simulink model "Thirtybussys"  (R2023b)
settings: Solver=VariableStepAuto  StartTime=0.0  StopTime=1  RelTol=1e-3
libraries: spsFourierLib x60, spsThreePhaseSeriesRLCBranchLib x41, spsThreePhaseVIMeasurementLib x30, spsPower3phInstantaneousLib x30, spsThreePhaseSeriesRLCLoadLib x21, spsThreePhaseSourceLib x6, spsThreePhaseTransformerTwoWindingsLib x6, spsThreePhaseFaultLib x1, sps_lib x1
(part 1 of 2)
settings Model: Creator=sariy sh  LastModifiedBy=HP
settings SolverCC: AlgebraicLoopSolver=TrustRegion
settings DataIOCC: ReturnWorkspaceOutputs=off
settings DebuggingCC: UnconnectedInputMsg=warning  UnconnectedOutputMsg=warning  UnconnectedLineMsg=warning  ArithmeticOperatorsInVariantConditions=warning
settings ModelReferenceCC: EnableRefExpFcnMdlSchedulingChecks=on
settings SFSimCC: SimUseLocalCustomCode=off  CustomCodeUndefinedFunction=UseInterfaceOnly
settings RTWCC: RTWUseLocalCustomCode=off
settings CodeAppCC: StateflowObjectComments=on
settings SimscapeCC: SimscapeNormalizeSystem=off

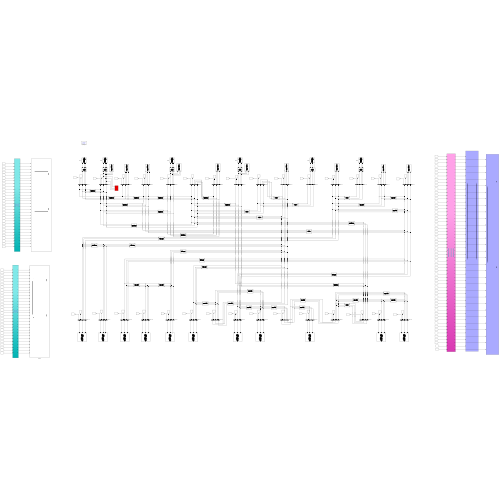
[thumbnail: Simulink's stored preview of the top-level diagram]
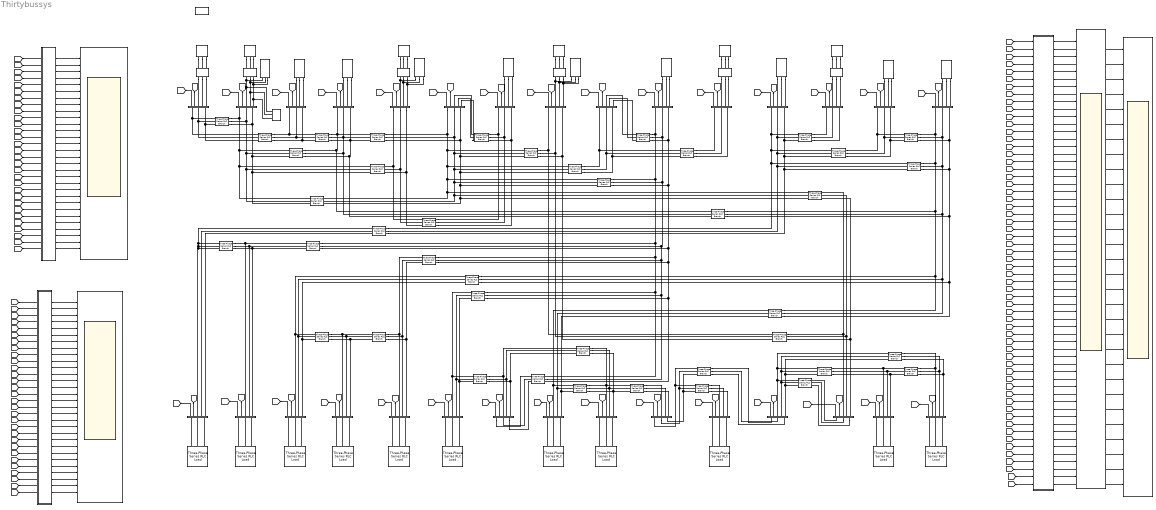
== system Thirtybussys ==
  Bus {1..30} (30 alike) : spsThreePhaseVIMeasurementLib/Three-Phase V-I Measurement  VoltageMeasurement=phase-to-ground  SetLabelV=off  LabelV=Vabc  Vpu=off  VpuLL=off  CurrentMeasurement=yes  SetLabelI=off  LabelI=Iabc  Ipu=off  Pbase=100e6  Vbase=500e3  OutputType=Complex  PhasorSimulation=off  PSBequivalent=0
  Gen1 : spsThreePhaseSourceLib/Three-Phase Source  InternalConnection=Yg  VoltagePhases=off  Voltage=1.06  PhaseAngle=0  Voltage_phases=[25e3 25e3 25e3]/sqrt(3)  PhaseAngles_phases=[0 -120 +120]  Frequency=50  NonIdealSource=on  SpecifyImpedance=on  Resistance=0.8929  Inductance=16.58e-3  ShortCircuitLevel=100e6  BaseVoltage=1  XRratio=1  BusType=swing  Pref=10e3  Qref=0  Prefabc=[10e3, 10e3, 10e3]  Qrefabc=[0, 0, 0]  Qmin=-inf  Qmax=inf
  Gen2 : spsThreePhaseSourceLib/Three-Phase Source  InternalConnection=Yg  VoltagePhases=off  Voltage=1.045  PhaseAngle=0  Voltage_phases=[25e3 25e3 25e3]/sqrt(3)  PhaseAngles_phases=[0 -120 +120]  Frequency=50  NonIdealSource=on  SpecifyImpedance=on  Resistance=0.8929  Inductance=16.58e-3  ShortCircuitLevel=100e6  BaseVoltage=1  XRratio=1  BusType=PQ  Pref=0.4  Qref=0.5  Prefabc=[10e3, 10e3, 10e3]  Qrefabc=[0, 0, 0]  Qmin=-inf  Qmax=inf
  Gen3 : spsThreePhaseSourceLib/Three-Phase Source  InternalConnection=Yg  VoltagePhases=off  Voltage=1.010  PhaseAngle=0  Voltage_phases=[25e3 25e3 25e3]/sqrt(3)  PhaseAngles_phases=[0 -120 +120]  Frequency=50  NonIdealSource=on  SpecifyImpedance=on  Resistance=0.8929  Inductance=16.58e-3  ShortCircuitLevel=100e6  BaseVoltage=1  XRratio=1  BusType=PV  Pref=0.37  Qref=0  Prefabc=[10e3, 10e3, 10e3]  Qrefabc=[0, 0, 0]  Qmin=-0.15  Qmax=0.625
  Gen4 : spsThreePhaseSourceLib/Three-Phase Source  InternalConnection=Yg  VoltagePhases=off  Voltage=1.010  PhaseAngle=0  Voltage_phases=[25e3 25e3 25e3]/sqrt(3)  PhaseAngles_phases=[0 -120 +120]  Frequency=50  NonIdealSource=on  SpecifyImpedance=on  Resistance=0.8929  Inductance=16.58e-3  ShortCircuitLevel=100e6  BaseVoltage=1  XRratio=1  BusType=PV  Pref=0.373  Qref=0  Prefabc=[10e3, 10e3, 10e3]  Qrefabc=[0, 0, 0]  Qmin=-0.15  Qmax=0.50
  Gen5 : spsThreePhaseSourceLib/Three-Phase Source  InternalConnection=Yg  VoltagePhases=off  Voltage=1.082  PhaseAngle=0  Voltage_phases=[25e3 25e3 25e3]/sqrt(3)  PhaseAngles_phases=[0 -120 +120]  Frequency=50  NonIdealSource=on  SpecifyImpedance=on  Resistance=0.8929  Inductance=16.58e-3  ShortCircuitLevel=100e6  BaseVoltage=1  XRratio=1  BusType=PV  Pref=0.162  Qref=0  Prefabc=[10e3, 10e3, 10e3]  Qrefabc=[0, 0, 0]  Qmin=-0.10  Qmax=0.40
  Gen6 : spsThreePhaseSourceLib/Three-Phase Source  InternalConnection=Yg  VoltagePhases=off  Voltage=1.071  PhaseAngle=0  Voltage_phases=[25e3 25e3 25e3]/sqrt(3)  PhaseAngles_phases=[0 -120 +120]  Frequency=50  NonIdealSource=on  SpecifyImpedance=on  Resistance=0.8929  Inductance=16.58e-3  ShortCircuitLevel=100e6  BaseVoltage=1  XRratio=1  BusType=PV  Pref=0.106  Qref=0  Prefabc=[10e3, 10e3, 10e3]  Qrefabc=[0, 0, 0]  Qmin=-0.15  Qmax=0.45
  Scope{,1..3} (4 alike) : Scope  NumInputPorts=30
  Subsystem : Subsystem
  Subsystem1 : Subsystem
  Subsystem30 : Subsystem
  Three-Phase Series RLC Branch : spsThreePhaseSeriesRLCBranchLib/Three-Phase Series RLC Branch  LConnTagsString=A|B|C  RConnTagsString=A|B|C  BranchType=RLC  Resistance=0.0192  Inductance=0.0575/(2*pi*50)  Capacitance=1/0.0264/(2*pi*50)  Measurements=None
  Three-Phase Series RLC Branch1 : spsThreePhaseSeriesRLCBranchLib/Three-Phase Series RLC Branch  LConnTagsString=A|B|C  RConnTagsString=A|B|C  BranchType=RLC  Resistance=0.0452  Inductance=0.1652/(2*pi*50)  Capacitance=1/0.0204/(2*pi*50)  Measurements=None
  Three-Phase Series RLC Branch10 : spsThreePhaseSeriesRLCBranchLib/Three-Phase Series RLC Branch  LConnTagsString=A|B|C  RConnTagsString=A|B|C  BranchType=L  Resistance=0  Inductance=0.2080/(2*pi*50)  Capacitance=0  Measurements=None
  Three-Phase Series RLC Branch11 : spsThreePhaseSeriesRLCBranchLib/Three-Phase Series RLC Branch  LConnTagsString=A|B|C  RConnTagsString=A|B|C  BranchType=L  Resistance=1  Inductance=0.1100/(2*pi*50)  Capacitance=1e-6  Measurements=None
  Three-Phase Series RLC Branch12 : spsThreePhaseSeriesRLCBranchLib/Three-Phase Series RLC Branch  LConnTagsString=A|B|C  RConnTagsString=A|B|C  BranchType=L  Resistance=1  Inductance=0.5560/(2*pi*50)  Capacitance=1e-6  Measurements=None
  Three-Phase Series RLC Branch13 : spsThreePhaseSeriesRLCBranchLib/Three-Phase Series RLC Branch  LConnTagsString=A|B|C  RConnTagsString=A|B|C  BranchType=L  Resistance=1  Inductance=0.2080/(2*pi*50)  Capacitance=1e-6  Measurements=None
  Three-Phase Series RLC Branch14 : spsThreePhaseSeriesRLCBranchLib/Three-Phase Series RLC Branch  LConnTagsString=A|B|C  RConnTagsString=A|B|C  BranchType=L  Resistance=1  Inductance=0.1400/(2*pi*50)  Capacitance=1e-6  Measurements=None
  Three-Phase Series RLC Branch15 : spsThreePhaseSeriesRLCBranchLib/Three-Phase Series RLC Branch  LConnTagsString=A|B|C  RConnTagsString=A|B|C  BranchType=RL  Resistance=0.1231  Inductance=0.2559/(2*pi*50)  Capacitance=1e-6  Measurements=None
  Three-Phase Series RLC Branch16 : spsThreePhaseSeriesRLCBranchLib/Three-Phase Series RLC Branch  LConnTagsString=A|B|C  RConnTagsString=A|B|C  BranchType=RL  Resistance=0.2210  Inductance=0.1997/(2*pi*50)  Capacitance=1e-6  Measurements=None
  Three-Phase Series RLC Branch17 : spsThreePhaseSeriesRLCBranchLib/Three-Phase Series RLC Branch  LConnTagsString=A|B|C  RConnTagsString=A|B|C  BranchType=L  Resistance=1  Inductance=0.2560/(2*pi*50)  Capacitance=1e-6  Measurements=None
  Three-Phase Series RLC Branch18 : spsThreePhaseSeriesRLCBranchLib/Three-Phase Series RLC Branch  LConnTagsString=A|B|C  RConnTagsString=A|B|C  BranchType=RL  Resistance=0.0945  Inductance=0.1987/(2*pi*50)  Capacitance=1e-6  Measurements=None
  Three-Phase Series RLC Branch19 : spsThreePhaseSeriesRLCBranchLib/Three-Phase Series RLC Branch  LConnTagsString=A|B|C  RConnTagsString=A|B|C  BranchType=RLC  Resistance=0.0524  Inductance=0.1923/(2*pi*50)  Capacitance=1e-6  Measurements=None
  Three-Phase Series RLC Branch2 : spsThreePhaseSeriesRLCBranchLib/Three-Phase Series RLC Branch  LConnTagsString=A|B|C  RConnTagsString=A|B|C  BranchType=RLC  Resistance=0.0132  Inductance=0.0379/(2*pi*50)  Capacitance=1/0.0042/(2*pi*50)  Measurements=None
  Three-Phase Series RLC Branch20 : spsThreePhaseSeriesRLCBranchLib/Three-Phase Series RLC Branch  LConnTagsString=A|B|C  RConnTagsString=A|B|C  BranchType=RL  Resistance=0.0324  Inductance=0.0845/(2*pi*50)  Capacitance=1e-6  Measurements=None
  Three-Phase Series RLC Branch21 : spsThreePhaseSeriesRLCBranchLib/Three-Phase Series RLC Branch  LConnTagsString=A|B|C  RConnTagsString=A|B|C  BranchType=RL  Resistance=0.1063  Inductance=0.2185/(2*pi*50)  Capacitance=1e-6  Measurements=None
  Three-Phase Series RLC Branch22 : spsThreePhaseSeriesRLCBranchLib/Three-Phase Series RLC Branch  LConnTagsString=A|B|C  RConnTagsString=A|B|C  BranchType=RL  Resistance=0.0639  Inductance=0.1292/(2*pi*50)  Capacitance=1e-6  Measurements=None
  Three-Phase Series RLC Branch23 : spsThreePhaseSeriesRLCBranchLib/Three-Phase Series RLC Branch  LConnTagsString=A|B|C  RConnTagsString=A|B|C  BranchType=RL  Resistance=0.0340  Inductance=0.0680/(2*pi*50)  Capacitance=1e-6  Measurements=None
  Three-Phase Series RLC Branch24 : spsThreePhaseSeriesRLCBranchLib/Three-Phase Series RLC Branch  LConnTagsString=A|B|C  RConnTagsString=A|B|C  BranchType=RL  Resistance=0.0936  Inductance=0.2090/(2*pi*50)  Capacitance=1e-6  Measurements=None
  Three-Phase Series RLC Branch25 : spsThreePhaseSeriesRLCBranchLib/Three-Phase Series RLC Branch  LConnTagsString=A|B|C  RConnTagsString=A|B|C  BranchType=RL  Resistance=0.0348  Inductance=0.0749/(2*pi*50)  Capacitance=1e-6  Measurements=None
  Three-Phase Series RLC Branch26 : spsThreePhaseSeriesRLCBranchLib/Three-Phase Series RLC Branch  LConnTagsString=A|B|C  RConnTagsString=A|B|C  BranchType=RL  Resistance=0.0116  Inductance=0.0236/(2*pi*50)  Capacitance=1e-6  Measurements=None
  Three-Phase Series RLC Branch27 : spsThreePhaseSeriesRLCBranchLib/Three-Phase Series RLC Branch  LConnTagsString=A|B|C  RConnTagsString=A|B|C  BranchType=RL  Resistance=0.0727  Inductance=0.1499/(2*pi*50)  Capacitance=1e-6  Measurements=None
  Three-Phase Series RLC Branch28 : spsThreePhaseSeriesRLCBranchLib/Three-Phase Series RLC Branch  LConnTagsString=A|B|C  RConnTagsString=A|B|C  BranchType=RL  Resistance=0.1000  Inductance=0.2020/(2*pi*50)  Capacitance=1e-6  Measurements=None
  Three-Phase Series RLC Branch29 : spsThreePhaseSeriesRLCBranchLib/Three-Phase Series RLC Branch  LConnTagsString=A|B|C  RConnTagsString=A|B|C  BranchType=RL  Resistance=0.1150  Inductance=0.1790/(2*pi*50)  Capacitance=1e-6  Measurements=None
  Three-Phase Series RLC Branch3 : spsThreePhaseSeriesRLCBranchLib/Three-Phase Series RLC Branch  LConnTagsString=A|B|C  RConnTagsString=A|B|C  BranchType=RLC  Resistance=0.0570  Inductance=0.1737/(2*pi*50)  Capacitance=1/0.0184/(2*pi*50)  Measurements=None
  Three-Phase Series RLC Branch30 : spsThreePhaseSeriesRLCBranchLib/Three-Phase Series RLC Branch  LConnTagsString=A|B|C  RConnTagsString=A|B|C  BranchType=RL  Resistance=0.1320  Inductance=0.2700/(2*pi*50)  Capacitance=1e-6  Measurements=None
  Three-Phase Series RLC Branch31 : spsThreePhaseSeriesRLCBranchLib/Three-Phase Series RLC Branch  LConnTagsString=A|B|C  RConnTagsString=A|B|C  BranchType=RL  Resistance=0.1885  Inductance=0.3292/(2*pi*50)  Capacitance=1e-6  Measurements=None
  Three-Phase Series RLC Branch32 : spsThreePhaseSeriesRLCBranchLib/Three-Phase Series RLC Branch  LConnTagsString=A|B|C  RConnTagsString=A|B|C  BranchType=RL  Resistance=0.2544  Inductance=0.3800/(2*pi*50)  Capacitance=1e-6  Measurements=None
  Three-Phase Series RLC Branch33 : spsThreePhaseSeriesRLCBranchLib/Three-Phase Series RLC Branch  LConnTagsString=A|B|C  RConnTagsString=A|B|C  BranchType=RL  Resistance=0.1093  Inductance=0.2087/(2*pi*50)  Capacitance=1e-6  Measurements=None
  Three-Phase Series RLC Branch34 : spsThreePhaseSeriesRLCBranchLib/Three-Phase Series RLC Branch  LConnTagsString=A|B|C  RConnTagsString=A|B|C  BranchType=RL  Resistance=0.2198  Inductance=0.4153/(2*pi*50)  Capacitance=1e-6  Measurements=None
  Three-Phase Series RLC Branch35 : spsThreePhaseSeriesRLCBranchLib/Three-Phase Series RLC Branch  LConnTagsString=A|B|C  RConnTagsString=A|B|C  BranchType=RL  Resistance=0.3202  Inductance=0.6027/(2*pi*50)  Capacitance=1e-6  Measurements=None
  Three-Phase Series RLC Branch36 : spsThreePhaseSeriesRLCBranchLib/Three-Phase Series RLC Branch  LConnTagsString=A|B|C  RConnTagsString=A|B|C  BranchType=L  Resistance=1  Inductance=0.3960/(2*pi*50)  Capacitance=1e-6  Measurements=None
  Three-Phase Series RLC Branch37 : spsThreePhaseSeriesRLCBranchLib/Three-Phase Series RLC Branch  LConnTagsString=A|B|C  RConnTagsString=A|B|C  BranchType=RLC  Resistance=0.0169  Inductance=0.0599/(2*pi*50)  Capacitance=1/0.0065/(2*pi*50)  Measurements=None
  Three-Phase Series RLC Branch38 : spsThreePhaseSeriesRLCBranchLib/Three-Phase Series RLC Branch  LConnTagsString=A|B|C  RConnTagsString=A|B|C  BranchType=RLC  Resistance=0.0636  Inductance=0.2000/(2*pi*50)  Capacitance=1/0.0214/(2*pi*50)  Measurements=None
  Three-Phase Series RLC Branch39 : spsThreePhaseSeriesRLCBranchLib/Three-Phase Series RLC Branch  LConnTagsString=A|B|C  RConnTagsString=A|B|C  BranchType=RL  Resistance=0.0662  Inductance=0.1304/(2*pi*50)  Capacitance=1e-6  Measurements=None
  Three-Phase Series RLC Branch4 : spsThreePhaseSeriesRLCBranchLib/Three-Phase Series RLC Branch  LConnTagsString=A|B|C  RConnTagsString=A|B|C  BranchType=RLC  Resistance=0.0472  Inductance=0.1983/(2*pi*50)  Capacitance=1/0.0209/(2*pi*50)  Measurements=None
  Three-Phase Series RLC Branch40 : spsThreePhaseSeriesRLCBranchLib/Three-Phase Series RLC Branch  LConnTagsString=A|B|C  RConnTagsString=A|B|C  BranchType=RL  Resistance=0.2399  Inductance=0.4533/(2*pi*50)  Capacitance=1e-6  Measurements=None
  Three-Phase Series RLC Branch5 : spsThreePhaseSeriesRLCBranchLib/Three-Phase Series RLC Branch  LConnTagsString=A|B|C  RConnTagsString=A|B|C  BranchType=RLC  Resistance=0.0581  Inductance=0.1763/(2*pi*50)  Capacitance=1/0.0187/(2*pi*50)  Measurements=None
  Three-Phase Series RLC Branch6 : spsThreePhaseSeriesRLCBranchLib/Three-Phase Series RLC Branch  LConnTagsString=A|B|C  RConnTagsString=A|B|C  BranchType=RLC  Resistance=0.0119  Inductance=0.0414/(2*pi*50)  Capacitance=1/0.0045/(2*pi*50)  Measurements=None
  Three-Phase Series RLC Branch7 : spsThreePhaseSeriesRLCBranchLib/Three-Phase Series RLC Branch  LConnTagsString=A|B|C  RConnTagsString=A|B|C  BranchType=RLC  Resistance=0.0267  Inductance=0.0820/(2*pi*50)  Capacitance=1/0.0085/(2*pi*50)  Measurements=None
  Three-Phase Series RLC Branch8 : spsThreePhaseSeriesRLCBranchLib/Three-Phase Series RLC Branch  LConnTagsString=A|B|C  RConnTagsString=A|B|C  BranchType=RLC  Resistance=0.0460  Inductance=0.1160/(2*pi*50)  Capacitance=1/0.0102/(2*pi*50)  Measurements=None
  Three-Phase Series RLC Branch9 : spsThreePhaseSeriesRLCBranchLib/Three-Phase Series RLC Branch  LConnTagsString=A|B|C  RConnTagsString=A|B|C  BranchType=RLC  Resistance=0.0120  Inductance=0.0420/(2*pi*50)  Capacitance=1/0.0045/(2*pi*50)  Measurements=None
  Three-Phase Series RLC Load : spsThreePhaseSeriesRLCLoadLib/Three-Phase Series RLC Load  LConnTagsString=A|B|C  Configuration=Y (grounded)  NominalVoltage=1  Vabc=[1e3 1e3 1e3]  Vabcp=[1e3 1e3 1e3]  NominalFrequency=50  UnbalancedPower=off  ActivePower=0.217  InductivePower=0.127  CapacitivePower=0  Pabc=[10e3 9e3 11e3]  QLabc=[100 90 110]  QCabc=[100 90 110]  Pabcp=[10e3 9e3 11e3]  QLabcp=[100 90 110]  QCabcp=[100 90 110]  Measurements=None  LoadType=constant Z
  Three-Phase Series RLC Load1 : spsThreePhaseSeriesRLCLoadLib/Three-Phase Series RLC Load  LConnTagsString=A|B|C  Configuration=Y (grounded)  NominalVoltage=1  Vabc=[1e3 1e3 1e3]  Vabcp=[1e3 1e3 1e3]  NominalFrequency=50  UnbalancedPower=off  ActivePower=0.024  InductivePower=0.012  CapacitivePower=0  Pabc=[10e3 9e3 11e3]  QLabc=[100 90 110]  QCabc=[100 90 110]  Pabcp=[10e3 9e3 11e3]  QLabcp=[100 90 110]  QCabcp=[100 90 110]  Measurements=None  LoadType=constant Z
  Three-Phase Series RLC Load10 : spsThreePhaseSeriesRLCLoadLib/Three-Phase Series RLC Load  LConnTagsString=A|B|C  Configuration=Y (grounded)  NominalVoltage=1  Vabc=[1e3 1e3 1e3]  Vabcp=[1e3 1e3 1e3]  NominalFrequency=50  UnbalancedPower=off  ActivePower=0.062  InductivePower=0.016  CapacitivePower=0  Pabc=[10e3 9e3 11e3]  QLabc=[100 90 110]  QCabc=[100 90 110]  Pabcp=[10e3 9e3 11e3]  QLabcp=[100 90 110]  QCabcp=[100 90 110]  Measurements=None  LoadType=constant Z
  Three-Phase Series RLC Load11 : spsThreePhaseSeriesRLCLoadLib/Three-Phase Series RLC Load  LConnTagsString=A|B|C  Configuration=Y (grounded)  NominalVoltage=1  Vabc=[1e3 1e3 1e3]  Vabcp=[1e3 1e3 1e3]  NominalFrequency=50  UnbalancedPower=off  ActivePower=0.082  InductivePower=0.025  CapacitivePower=0  Pabc=[10e3 9e3 11e3]  QLabc=[100 90 110]  QCabc=[100 90 110]  Pabcp=[10e3 9e3 11e3]  QLabcp=[100 90 110]  QCabcp=[100 90 110]  Measurements=None  LoadType=constant Z
  Three-Phase Series RLC Load12 : spsThreePhaseSeriesRLCLoadLib/Three-Phase Series RLC Load  LConnTagsString=A|B|C  Configuration=Y (grounded)  NominalVoltage=1  Vabc=[1e3 1e3 1e3]  Vabcp=[1e3 1e3 1e3]  NominalFrequency=50  UnbalancedPower=off  ActivePower=0.3  InductivePower=0.3  CapacitivePower=0  Pabc=[10e3 9e3 11e3]  QLabc=[100 90 110]  QCabc=[100 90 110]  Pabcp=[10e3 9e3 11e3]  QLabcp=[100 90 110]  QCabcp=[100 90 110]  Measurements=None  LoadType=constant Z
  Three-Phase Series RLC Load13 : spsThreePhaseSeriesRLCLoadLib/Three-Phase Series RLC Load  LConnTagsString=A|B|C  Configuration=Y (grounded)  NominalVoltage=1  Vabc=[1e3 1e3 1e3]  Vabcp=[1e3 1e3 1e3]  NominalFrequency=50  UnbalancedPower=off  ActivePower=0.032  InductivePower=0.009  CapacitivePower=0  Pabc=[10e3 9e3 11e3]  QLabc=[100 90 110]  QCabc=[100 90 110]  Pabcp=[10e3 9e3 11e3]  QLabcp=[100 90 110]  QCabcp=[100 90 110]  Measurements=None  LoadType=constant Z
  Three-Phase Series RLC Load14 : spsThreePhaseSeriesRLCLoadLib/Three-Phase Series RLC Load  LConnTagsString=A|B|C  Configuration=Y (grounded)  NominalVoltage=1  Vabc=[1e3 1e3 1e3]  Vabcp=[1e3 1e3 1e3]  NominalFrequency=50  UnbalancedPower=off  ActivePower=0.095  InductivePower=0.034  CapacitivePower=0  Pabc=[10e3 9e3 11e3]  QLabc=[100 90 110]  QCabc=[100 90 110]  Pabcp=[10e3 9e3 11e3]  QLabcp=[100 90 110]  QCabcp=[100 90 110]  Measurements=None  LoadType=constant Z
  Three-Phase Series RLC Load15 : spsThreePhaseSeriesRLCLoadLib/Three-Phase Series RLC Load  LConnTagsString=A|B|C  Configuration=Y (grounded)  NominalVoltage=1  Vabc=[1e3 1e3 1e3]  Vabcp=[1e3 1e3 1e3]  NominalFrequency=50  UnbalancedPower=off  ActivePower=0.022  InductivePower=0.007  CapacitivePower=0  Pabc=[10e3 9e3 11e3]  QLabc=[100 90 110]  QCabc=[100 90 110]  Pabcp=[10e3 9e3 11e3]  QLabcp=[100 90 110]  QCabcp=[100 90 110]  Measurements=None  LoadType=constant Z
  Three-Phase Series RLC Load16 : spsThreePhaseSeriesRLCLoadLib/Three-Phase Series RLC Load  LConnTagsString=A|B|C  Configuration=Y (grounded)  NominalVoltage=1  Vabc=[1e3 1e3 1e3]  Vabcp=[1e3 1e3 1e3]  NominalFrequency=50  UnbalancedPower=off  ActivePower=0.175  InductivePower=0.112  CapacitivePower=0  Pabc=[10e3 9e3 11e3]  QLabc=[100 90 110]  QCabc=[100 90 110]  Pabcp=[10e3 9e3 11e3]  QLabcp=[100 90 110]  QCabcp=[100 90 110]  Measurements=None  LoadType=constant Z
  Three-Phase Series RLC Load17 : spsThreePhaseSeriesRLCLoadLib/Three-Phase Series RLC Load  LConnTagsString=A|B|C  Configuration=Y (grounded)  NominalVoltage=1  Vabc=[1e3 1e3 1e3]  Vabcp=[1e3 1e3 1e3]  NominalFrequency=50  UnbalancedPower=off  ActivePower=0.032  InductivePower=0.016  CapacitivePower=0  Pabc=[10e3 9e3 11e3]  QLabc=[100 90 110]  QCabc=[100 90 110]  Pabcp=[10e3 9e3 11e3]  QLabcp=[100 90 110]  QCabcp=[100 90 110]  Measurements=None  LoadType=constant Z
  Three-Phase Series RLC Load18 : spsThreePhaseSeriesRLCLoadLib/Three-Phase Series RLC Load  LConnTagsString=A|B|C  Configuration=Y (grounded)  NominalVoltage=1  Vabc=[1e3 1e3 1e3]  Vabcp=[1e3 1e3 1e3]  NominalFrequency=50  UnbalancedPower=off  ActivePower=0.087  InductivePower=0.067  CapacitivePower=0  Pabc=[10e3 9e3 11e3]  QLabc=[100 90 110]  QCabc=[100 90 110]  Pabcp=[10e3 9e3 11e3]  QLabcp=[100 90 110]  QCabcp=[100 90 110]  Measurements=None  LoadType=constant Z
  Three-Phase Series RLC Load19 : spsThreePhaseSeriesRLCLoadLib/Three-Phase Series RLC Load  LConnTagsString=A|B|C  Configuration=Y (grounded)  NominalVoltage=1  Vabc=[1e3 1e3 1e3]  Vabcp=[1e3 1e3 1e3]  NominalFrequency=50  UnbalancedPower=off  ActivePower=0.035  InductivePower=0.023  CapacitivePower=0  Pabc=[10e3 9e3 11e3]  QLabc=[100 90 110]  QCabc=[100 90 110]  Pabcp=[10e3 9e3 11e3]  QLabcp=[100 90 110]  QCabcp=[100 90 110]  Measurements=None  LoadType=constant Z
  Three-Phase Series RLC Load2 : spsThreePhaseSeriesRLCLoadLib/Three-Phase Series RLC Load  LConnTagsString=A|B|C  Configuration=Y (grounded)  NominalVoltage=1  Vabc=[1e3 1e3 1e3]  Vabcp=[1e3 1e3 1e3]  NominalFrequency=50  UnbalancedPower=off  ActivePower=0.076  InductivePower=0.016  CapacitivePower=0  Pabc=[10e3 9e3 11e3]  QLabc=[100 90 110]  QCabc=[100 90 110]  Pabcp=[10e3 9e3 11e3]  QLabcp=[100 90 110]  QCabcp=[100 90 110]  Measurements=None  LoadType=constant Z
  Three-Phase Series RLC Load21 : spsThreePhaseSeriesRLCLoadLib/Three-Phase Series RLC Load  LConnTagsString=A|B|C  Configuration=Y (grounded)  NominalVoltage=1  Vabc=[1e3 1e3 1e3]  Vabcp=[1e3 1e3 1e3]  NominalFrequency=50  UnbalancedPower=off  ActivePower=0.024  InductivePower=0.009  CapacitivePower=0  Pabc=[10e3 9e3 11e3]  QLabc=[100 90 110]  QCabc=[100 90 110]  Pabcp=[10e3 9e3 11e3]  QLabcp=[100 90 110]  QCabcp=[100 90 110]  Measurements=None  LoadType=constant Z
  Three-Phase Series RLC Load22 : spsThreePhaseSeriesRLCLoadLib/Three-Phase Series RLC Load  LConnTagsString=A|B|C  Configuration=Y (grounded)  NominalVoltage=1  Vabc=[1e3 1e3 1e3]  Vabcp=[1e3 1e3 1e3]  NominalFrequency=50  UnbalancedPower=off  ActivePower=0.106  InductivePower=0.019  CapacitivePower=0  Pabc=[10e3 9e3 11e3]  QLabc=[100 90 110]  QCabc=[100 90 110]  Pabcp=[10e3 9e3 11e3]  QLabcp=[100 90 110]  QCabcp=[100 90 110]  Measurements=None  LoadType=constant Z
  Three-Phase Series RLC Load3 : spsThreePhaseSeriesRLCLoadLib/Three-Phase Series RLC Load  LConnTagsString=A|B|C  Configuration=Y (grounded)  NominalVoltage=1  Vabc=[1e3 1e3 1e3]  Vabcp=[1e3 1e3 1e3]  NominalFrequency=50  UnbalancedPower=off  ActivePower=0.942  InductivePower=0.19  CapacitivePower=0  Pabc=[10e3 9e3 11e3]  QLabc=[100 90 110]  QCabc=[100 90 110]  Pabcp=[10e3 9e3 11e3]  QLabcp=[100 90 110]  QCabcp=[100 90 110]  Measurements=None  LoadType=constant Z
  Three-Phase Series RLC Load5 : spsThreePhaseSeriesRLCLoadLib/Three-Phase Series RLC Load  LConnTagsString=A|B|C  Configuration=Y (grounded)  NominalVoltage=1  Vabc=[1e3 1e3 1e3]  Vabcp=[1e3 1e3 1e3]  NominalFrequency=50  UnbalancedPower=off  ActivePower=0.228  InductivePower=0.109  CapacitivePower=0  Pabc=[10e3 9e3 11e3]  QLabc=[100 90 110]  QCabc=[100 90 110]  Pabcp=[10e3 9e3 11e3]  QLabcp=[100 90 110]  QCabcp=[100 90 110]  Measurements=None  LoadType=constant Z
  Three-Phase Series RLC Load6 : spsThreePhaseSeriesRLCLoadLib/Three-Phase Series RLC Load  LConnTagsString=A|B|C  Configuration=Y (grounded)  NominalVoltage=1  Vabc=[1e3 1e3 1e3]  Vabcp=[1e3 1e3 1e3]  NominalFrequency=50  UnbalancedPower=off  ActivePower=0.035  InductivePower=0.018  CapacitivePower=0  Pabc=[10e3 9e3 11e3]  QLabc=[100 90 110]  QCabc=[100 90 110]  Pabcp=[10e3 9e3 11e3]  QLabcp=[100 90 110]  QCabcp=[100 90 110]  Measurements=None  LoadType=constant Z
  Three-Phase Series RLC Load7 : spsThreePhaseSeriesRLCLoadLib/Three-Phase Series RLC Load  LConnTagsString=A|B|C  Configuration=Y (grounded)  NominalVoltage=1  Vabc=[1e3 1e3 1e3]  Vabcp=[1e3 1e3 1e3]  NominalFrequency=50  UnbalancedPower=off  ActivePower=0.058  InductivePower=0.02  CapacitivePower=0  Pabc=[10e3 9e3 11e3]  QLabc=[100 90 110]  QCabc=[100 90 110]  Pabcp=[10e3 9e3 11e3]  QLabcp=[100 90 110]  QCabcp=[100 90 110]  Measurements=None  LoadType=constant Z
  Three-Phase Series RLC Load8 : spsThreePhaseSeriesRLCLoadLib/Three-Phase Series RLC Load  LConnTagsString=A|B|C  Configuration=Y (grounded)  NominalVoltage=1  Vabc=[1e3 1e3 1e3]  Vabcp=[1e3 1e3 1e3]  NominalFrequency=50  UnbalancedPower=off  ActivePower=0.09  InductivePower=0.058  CapacitivePower=0  Pabc=[10e3 9e3 11e3]  QLabc=[100 90 110]  QCabc=[100 90 110]  Pabcp=[10e3 9e3 11e3]  QLabcp=[100 90 110]  QCabcp=[100 90 110]  Measurements=None  LoadType=constant Z
  Three-Phase Series RLC Load9 : spsThreePhaseSeriesRLCLoadLib/Three-Phase Series RLC Load  LConnTagsString=A|B|C  Configuration=Y (grounded)  NominalVoltage=1  Vabc=[1e3 1e3 1e3]  Vabcp=[1e3 1e3 1e3]  NominalFrequency=50  UnbalancedPower=off  ActivePower=0.112  InductivePower=0.075  CapacitivePower=0  Pabc=[10e3 9e3 11e3]  QLabc=[100 90 110]  QCabc=[100 90 110]  Pabcp=[10e3 9e3 11e3]  QLabcp=[100 90 110]  QCabcp=[100 90 110]  Measurements=None  LoadType=constant Z
  Three-Phase Transformer (Two Windings) : spsThreePhaseTransformerTwoWindingsLib/Three-Phase Transformer (Two Windings)  Winding1Connection=Yg  Winding2Connection=Yg  CoreType=Three single-phase transformers  SetSaturation=off  Hysteresis=off  DataFile='hysteresis'  SetInitialFlux=off  Measurements=None  UNITS=pu  NominalPower=[ 1 , 50 ]  Winding1=[1.06 , 0.002 , 0.08 ]  Winding2=[ 1.06 , 0.002 , 0.08 ]  Rm=500  Lm=500  L0=0.5  Saturation=[ 0,0 ; 0.0024,1.2 ; 1.0,1.52 ]  InitialFluxes=[ 0.8 , -0.8 , 0.7 ]  BreakLoop=off  DiscreteSolver=Trapezoidal iterative  DataType=off  TransfoNumber=1
  Three-Phase Transformer (Two Windings)1 : spsThreePhaseTransformerTwoWindingsLib/Three-Phase Transformer (Two Windings)  Winding1Connection=Yg  Winding2Connection=Yg  CoreType=Three single-phase transformers  SetSaturation=off  Hysteresis=off  DataFile='hysteresis'  SetInitialFlux=off  Measurements=None  UNITS=pu  NominalPower=[1 , 50 ]  Winding1=[ 1.045 , 0.002 , 0.08 ]  Winding2=[ 1.045 , 0.002 , 0.08 ]  Rm=500  Lm=500  L0=0.5  Saturation=[ 0,0 ; 0.0024,1.2 ; 1.0,1.52 ]  InitialFluxes=[ 0.8 , -0.8 , 0.7 ]  BreakLoop=off  DiscreteSolver=Trapezoidal iterative  DataType=off  TransfoNumber=1
  Three-Phase Transformer (Two Windings)2 : spsThreePhaseTransformerTwoWindingsLib/Three-Phase Transformer (Two Windings)  Winding1Connection=Yg  Winding2Connection=Yg  CoreType=Three single-phase transformers  SetSaturation=off  Hysteresis=off  DataFile='hysteresis'  SetInitialFlux=off  Measurements=None  UNITS=pu  NominalPower=[ 1 , 50 ]  Winding1=[ 1.010 , 0.002 , 0.08 ]  Winding2=[ 1.010 , 0.002 , 0.08 ]  Rm=500  Lm=500  L0=0.5  Saturation=[ 0,0 ; 0.0024,1.2 ; 1.0,1.52 ]  InitialFluxes=[ 0.8 , -0.8 , 0.7 ]  BreakLoop=off  DiscreteSolver=Trapezoidal iterative  DataType=off  TransfoNumber=1
  Three-Phase Transformer (Two Windings)3 : spsThreePhaseTransformerTwoWindingsLib/Three-Phase Transformer (Two Windings)  Winding1Connection=Yg  Winding2Connection=Yg  CoreType=Three single-phase transformers  SetSaturation=off  Hysteresis=off  DataFile='hysteresis'  SetInitialFlux=off  Measurements=None  UNITS=pu  NominalPower=[ 250e6 , 60 ]  Winding1=[ 735e3 , 0.002 , 0.08 ]  Winding2=[ 315e3 , 0.002 , 0.08 ]  Rm=500  Lm=500  L0=0.5  Saturation=[ 0,0 ; 0.0024,1.2 ; 1.0,1.52 ]  InitialFluxes=[ 0.8 , -0.8 , 0.7 ]  BreakLoop=off  DiscreteSolver=Trapezoidal iterative  DataType=off  TransfoNumber=1
  Three-Phase Transformer (Two Windings)4 : spsThreePhaseTransformerTwoWindingsLib/Three-Phase Transformer (Two Windings)  Winding1Connection=Yg  Winding2Connection=Yg  CoreType=Three single-phase transformers  SetSaturation=off  Hysteresis=off  DataFile='hysteresis'  SetInitialFlux=off  Measurements=None  UNITS=pu  NominalPower=[ 1 , 50 ]  Winding1=[ 1.082 , 0.002 , 0.08 ]  Winding2=[ 1.082 , 0.002 , 0.08 ]  Rm=500  Lm=500  L0=0.5  Saturation=[ 0,0 ; 0.0024,1.2 ; 1.0,1.52 ]  InitialFluxes=[ 0.8 , -0.8 , 0.7 ]  BreakLoop=off  DiscreteSolver=Trapezoidal iterative  DataType=off  TransfoNumber=1
  Three-Phase Transformer (Two Windings)5 : spsThreePhaseTransformerTwoWindingsLib/Three-Phase Transformer (Two Windings)  Winding1Connection=Yg  Winding2Connection=Yg  CoreType=Three single-phase transformers  SetSaturation=off  Hysteresis=off  DataFile='hysteresis'  SetInitialFlux=off  Measurements=None  UNITS=pu  NominalPower=[ 1 , 50 ]  Winding1=[ 1.071 , 0.002 , 0.08 ]  Winding2=[ 1.071 , 0.002 , 0.08 ]  Rm=500  Lm=500  L0=0.5  Saturation=[ 0,0 ; 0.0024,1.2 ; 1.0,1.52 ]  InitialFluxes=[ 0.8 , -0.8 , 0.7 ]  BreakLoop=off  DiscreteSolver=Trapezoidal iterative  DataType=off  TransfoNumber=1
  Three-Phase Fault : spsThreePhaseFaultLib/Three-Phase Fault  InitialStates=0  FaultA=on  FaultB=on  FaultC=on  GroundFault=on  SwitchTimes="[0.4  0.5]"  External=off  SwitchStatus=NaN  FaultResistance=0.001  GroundResistance=0.01  SnubberResistance=1e6  SnubberCapacitance=inf  Measurements=None
  powergui : sps_lib/powergui  Priority=1  SimulationMode=Discrete  SampleTime=50e-6  frequency=60  Iterations=50  frequencyindice=50  Pbase=100e6  ErrMax=1e-4  UnitsV=kV  UnitsW=MW  buscounter=0  FunctionMessages=off  echomessages=off  EnableUseOfTLC=off  CurrentSourceSwitches=off  DisableSnubberDevices=off  DisableRonSwitches=off  DisableVfSwitches=off  DisplayEquations=off  AutomaticDiscreteSolvers=off  SolverType=Tustin/Backward Euler (TBE)  Interpol=off  ExternalGateDelay=off  methode=off  Ts=100  x0status=blocks  SPID=off  SwTol=0  HookPort=off  NonlinearTolerance=1e-4  nMaxIteration=100  ContinueOnMaxIteration=off  RestoreLinks=warning  ResistiveCurrentMeasurement=off  Frange=[0:2:500]  Ylog=off  Xlog=on  ShowGrid=off  save=off  variable=ZData  structure=0  ZoomFFT=off  StartTime=0.0  cycles=1  DisplayStyle=1  fundamental=60  FreqAxis=off  MaxFrequency=1000  frequencyindicesteady=1  RmsSteady=1  display=off
  wires:
  Bus 1/1 -> [v1]
  Bus 1/2 -> [i1]
  Bus 2/1 -> [v2]
  Bus 2/2 -> [i2]
  Bus 3/1 -> [v3]
  Bus 3/2 -> [i3]
  Bus 4/1 -> [v4]
  Bus 4/2 -> [i4]
  Bus 5/1 -> [v5]
  Bus 5/2 -> [i5]
  Bus 6/1 -> [v6]
  Bus 6/2 -> [i6]
  Bus 7/2 -> [i7]
  Bus 7/1 -> [v7]
  Bus 8/1 -> [v8]
  Bus 8/2 -> [i8]
  Bus 9/1 -> [v9]
  Bus 9/2 -> [i9]
  Bus 10/1 -> [v10]
  Bus 10/2 -> [i10]
  Bus 11/1 -> [v11]
  Bus 11/2 -> [i11]
  Bus 12/1 -> [v12]
  Bus 12/2 -> [i12]
  Bus 13/2 -> [i13]
  Bus 14/1 -> [v14]
  Bus 14/2 -> [i14]
  Bus 15/2 -> [i15]
  Bus 16/1 -> [v16]
  Bus 16/2 -> [i16]
  Bus 17/2 -> [i17]
  Bus 18/1 -> [v18]
  Bus 18/2 -> [i18]
  Bus 19/1 -> [v19]
  Bus 19/2 -> [i19]
  Bus 20/1 -> [v20]
  Bus 20/2 -> [i20]
  Bus 21/1 -> [v21]
  Bus 21/2 -> [i21]
  Bus 22/1 -> [v22]
  Bus 22/2 -> [i22]
  Bus 23/1 -> [v23]
  Bus 23/2 -> [i23]
  Bus 24/1 -> [v24]
  Bus 24/2 -> [i24]
  Bus 25/1 -> [v25]
  Bus 25/2 -> [i25]
  Bus 26/1 -> [v26]
  Bus 26/2 -> [i26]
  Bus 27/2 -> [i27]
  Bus 28/2 -> [i28]
  Bus 29/1 -> [v29]
  Bus 29/2 -> [i29]
  Bus 30/2 -> [i30]
  Subsystem30/1(Out1) -> Scope/1
  Subsystem30/2(Out2) -> Scope/2
  Subsystem30/3(Out3) -> Scope/3
  Subsystem30/4(Out4) -> Scope/4
  Subsystem30/5(Out5) -> Scope/5
  Subsystem30/6(Out6) -> Scope/6
  Subsystem30/7(Out7) -> Scope/7
  Subsystem30/8(Out8) -> Scope/8
  Subsystem30/9(Out9) -> Scope/9
  Subsystem30/10(Out10) -> Scope/10
  Subsystem30/11(Out11) -> Scope/11
  Subsystem30/12(Out12) -> Scope/12
  Subsystem30/13(Out13) -> Scope/13
  Subsystem30/14(Out14) -> Scope/14
  Subsystem30/15(Out15) -> Scope/15
  Subsystem30/16(Out16) -> Scope/16
  Subsystem30/17(Out17) -> Scope/17
  Subsystem30/18(Out18) -> Scope/18
  Subsystem30/19(Out19) -> Scope/19
  Subsystem30/20(Out20) -> Scope/20
  Subsystem30/21(Out21) -> Scope/21
  Subsystem30/22(Out22) -> Scope/22
  Subsystem30/23(Out23) -> Scope/23
  Subsystem30/24(Out24) -> Scope/24
  Subsystem30/25(Out25) -> Scope/25
  Subsystem30/26(Out26) -> Scope/26
  Subsystem30/27(Out27) -> Scope/27
  Subsystem30/28(Out28) -> Scope/28
  Subsystem30/30(Out30) -> Scope/30
  Subsystem30/29(Out29) -> Scope/29
  [v1] -> Subsystem30/1(In1)
  [v2] -> Subsystem30/2(In2)
  [v3] -> Subsystem30/3(In3)
  [v4] -> Subsystem30/4(In4)
  [v5] -> Subsystem30/5(In5)
  [v6] -> Subsystem30/6(In6)
  [v7] -> Subsystem30/7(In7)
  [v8] -> Subsystem30/8(In8)
  [v9] -> Subsystem30/9(In9)
  [v10] -> Subsystem30/10(In10)
  [v11] -> Subsystem30/11(In11)
  [v12] -> Subsystem30/12(In12)
  [v13] -> Subsystem30/13(In13)
  [v14] -> Subsystem30/14(In14)
  [v15] -> Subsystem30/15(In15)
  [v16] -> Subsystem30/16(In16)
  [v17] -> Subsystem30/17(In17)
  [v18] -> Subsystem30/18(In18)
  [v19] -> Subsystem30/19(In19)
  [v20] -> Subsystem30/20(In20)
  [v21] -> Subsystem30/21(In21)
  [v22] -> Subsystem30/22(In22)
  [v23] -> Subsystem30/23(In23)
  [v24] -> Subsystem30/24(In24)
  [v25] -> Subsystem30/25(In25)
  [v26] -> Subsystem30/26(In26)
  [v27] -> Subsystem30/27(In27)
  [v28] -> Subsystem30/28(In28)
  [v29] -> Subsystem30/29(In29)
  [v30] -> Subsystem30/30(In30)
  [i30] -> Subsystem1/30(In30)
  [i29] -> Subsystem1/29(In29)
  [i28] -> Subsystem1/28(In28)
  [i27] -> Subsystem1/27(In27)
  [i26] -> Subsystem1/26(In26)
  [i25] -> Subsystem1/25(In25)
  [i24] -> Subsystem1/24(In24)
  [i23] -> Subsystem1/23(In23)
  [i22] -> Subsystem1/22(In22)
  [i21] -> Subsystem1/21(In21)
  [i20] -> Subsystem1/20(In20)
  [i19] -> Subsystem1/19(In19)
  [i18] -> Subsystem1/18(In18)
  [i17] -> Subsystem1/17(In17)
  [i16] -> Subsystem1/16(In16)
  [i15] -> Subsystem1/15(In15)
  [i14] -> Subsystem1/14(In14)
  [i13] -> Subsystem1/13(In13)
  [i12] -> Subsystem1/12(In12)
  [i11] -> Subsystem1/11(In11)
  [i10] -> Subsystem1/10(In10)
  [i9] -> Subsystem1/9(In9)
  [i8] -> Subsystem1/8(In8)
  [i7] -> Subsystem1/7(In7)
  [i6] -> Subsystem1/6(In6)
  [i5] -> Subsystem1/5(In5)
  [i4] -> Subsystem1/4(In4)
  [i3] -> Subsystem1/3(In3)
  [i2] -> Subsystem1/2(In2)
  [i1] -> Subsystem1/1(In1)
  Subsystem1/29(Out29) -> Scope1/29
  Subsystem1/30(Out30) -> Scope1/30
  Subsystem1/28(Out28) -> Scope1/28
  Subsystem1/27(Out27) -> Scope1/27
  Subsystem1/26(Out26) -> Scope1/26
  Subsystem1/25(Out25) -> Scope1/25
  Subsystem1/24(Out24) -> Scope1/24
  Subsystem1/23(Out23) -> Scope1/23
  Subsystem1/22(Out22) -> Scope1/22
  Subsystem1/21(Out21) -> Scope1/21
  Subsystem1/20(Out20) -> Scope1/20
  Subsystem1/19(Out19) -> Scope1/19
  Subsystem1/18(Out18) -> Scope1/18
  Subsystem1/17(Out17) -> Scope1/17
  Subsystem1/16(Out16) -> Scope1/16
  Subsystem1/15(Out15) -> Scope1/15
  Subsystem1/14(Out14) -> Scope1/14
  Subsystem1/13(Out13) -> Scope1/13
  Subsystem1/12(Out12) -> Scope1/12
  Subsystem1/11(Out11) -> Scope1/11
  Subsystem1/10(Out10) -> Scope1/10
  Subsystem1/9(Out9) -> Scope1/9
  Subsystem1/8(Out8) -> Scope1/8
  Subsystem1/7(Out7) -> Scope1/7
  Subsystem1/6(Out6) -> Scope1/6
  Subsystem1/5(Out5) -> Scope1/5
  Subsystem1/4(Out4) -> Scope1/4
  Subsystem1/3(Out3) -> Scope1/3
  Subsystem1/2(Out2) -> Scope1/2
  Subsystem1/1(Out1) -> Scope1/1
  [v1] -> Subsystem/1(In1)
  [v2] -> Subsystem/3(In3)
  [v3] -> Subsystem/5(In5)
  [v5] -> Subsystem/9(In9)
  [v4] -> Subsystem/7(In7)
  [v6] -> Subsystem/11(In11)
  [v7] -> Subsystem/13(In13)
  [v8] -> Subsystem/15(In15)
  [v9] -> Subsystem/17(In17)
  [v11] -> Subsystem/21(In21)
  [v10] -> Subsystem/19(In19)
  [v12] -> Subsystem/23(In23)
  [v13] -> Subsystem/25(In25)
  [v14] -> Subsystem/27(In27)
  [v16] -> Subsystem/31(In31)
  [v15] -> Subsystem/29(In29)
  [v17] -> Subsystem/33(In33)
  [v18] -> Subsystem/35(In35)
  [v19] -> Subsystem/37(In37)
  [v20] -> Subsystem/39(In39)
  [v21] -> Subsystem/41(In41)
  [v22] -> Subsystem/43(In43)
  [v23] -> Subsystem/45(In45)
  [v24] -> Subsystem/47(In47)
  [v25] -> Subsystem/49(In49)
  [v26] -> Subsystem/51(In51)
  [v27] -> Subsystem/53(In53)
  [v28] -> Subsystem/55(In55)
  [v29] -> Subsystem/57(In57)
  [v30] -> Subsystem/59(In59)
  [i1] -> Subsystem/2(In2)
  [i2] -> Subsystem/4(In4)
  [i3] -> Subsystem/6(In6)
  [i4] -> Subsystem/8(In8)
  [i5] -> Subsystem/10(In10)
  [i6] -> Subsystem/12(In12)
  [i7] -> Subsystem/14(In14)
  [i8] -> Subsystem/16(In16)
  [i9] -> Subsystem/18(In18)
  [i10] -> Subsystem/20(In20)
  [i11] -> Subsystem/22(In22)
  [i12] -> Subsystem/24(In24)
  [i13] -> Subsystem/26(In26)
  [i14] -> Subsystem/28(In28)
  [i15] -> Subsystem/30(In30)
  [i16] -> Subsystem/32(In32)
  [i17] -> Subsystem/34(In34)
  [i18] -> Subsystem/36(In36)
  [i19] -> Subsystem/38(In38)
  [i20] -> Subsystem/40(In40)
  [i21] -> Subsystem/42(In42)
  [i22] -> Subsystem/44(In44)
  [i23] -> Subsystem/46(In46)
  [i25] -> Subsystem/50(In50)
  [i24] -> Subsystem/48(In48)
  [i26] -> Subsystem/52(In52)
  [i27] -> Subsystem/54(In54)
  [i28] -> Subsystem/56(In56)
  [i29] -> Subsystem/58(In58)
  [i30] -> Subsystem/60(In60)
  Subsystem/1(Out1) -> Scope2/1
  Subsystem/3(Out3) -> Scope2/2
  Subsystem/5(Out5) -> Scope2/3
  Subsystem/7(Out7) -> Scope2/4
  Subsystem/9(Out9) -> Scope2/5
  Subsystem/11(Out11) -> Scope2/6
  Subsystem/13(Out13) -> Scope2/7
  Subsystem/15(Out15) -> Scope2/8
  Subsystem/17(Out17) -> Scope2/9
  Subsystem/19(Out19) -> Scope2/10
  Subsystem/21(Out21) -> Scope2/11
  Subsystem/23(Out23) -> Scope2/12
  Subsystem/25(Out25) -> Scope2/13
  Subsystem/27(Out27) -> Scope2/14
  Subsystem/29(Out29) -> Scope2/15
  Subsystem/31(Out31) -> Scope2/16
  Subsystem/33(Out33) -> Scope2/17
  Subsystem/35(Out35) -> Scope2/18
  Subsystem/37(Out37) -> Scope2/19
  Subsystem/39(Out39) -> Scope2/20
  Subsystem/41(Out41) -> Scope2/21
  Subsystem/43(Out43) -> Scope2/22
  Subsystem/45(Out45) -> Scope2/23
  Subsystem/47(Out47) -> Scope2/24
  Subsystem/49(Out49) -> Scope2/25
  Subsystem/51(Out51) -> Scope2/26
  Subsystem/53(Out53) -> Scope2/27
  Subsystem/55(Out55) -> Scope2/28
  Subsystem/57(Out57) -> Scope2/29
  Subsystem/59(Out59) -> Scope2/30
  Subsystem/2(Out2) -> Scope3/1
  Subsystem/4(Out4) -> Scope3/2
  Subsystem/6(Out6) -> Scope3/3
  Subsystem/8(Out8) -> Scope3/4
  Subsystem/10(Out10) -> Scope3/5
  Subsystem/12(Out12) -> Scope3/6
  Subsystem/14(Out14) -> Scope3/7
  Subsystem/16(Out16) -> Scope3/8
  Subsystem/18(Out18) -> Scope3/9
  Subsystem/20(Out20) -> Scope3/10
  Subsystem/22(Out22) -> Scope3/11
  Subsystem/24(Out24) -> Scope3/12
  Subsystem/26(Out26) -> Scope3/13
  Subsystem/28(Out28) -> Scope3/14
  Subsystem/30(Out30) -> Scope3/15
  Subsystem/32(Out32) -> Scope3/16
  Subsystem/34(Out34) -> Scope3/17
  Subsystem/36(Out36) -> Scope3/18
  Subsystem/38(Out38) -> Scope3/19
  Subsystem/40(Out40) -> Scope3/20
  Subsystem/42(Out42) -> Scope3/21
  Subsystem/44(Out44) -> Scope3/22
  Subsystem/46(Out46) -> Scope3/23
  Subsystem/48(Out48) -> Scope3/24
  Subsystem/50(Out50) -> Scope3/25
  Subsystem/52(Out52) -> Scope3/26
  Subsystem/54(Out54) -> Scope3/27
  Subsystem/56(Out56) -> Scope3/28
  Subsystem/58(Out58) -> Scope3/29
  Subsystem/60(Out60) -> Scope3/30
  Bus 15/1 -> [v15]
  Bus 13/1 -> [v13]
  Bus 30/1 -> [v30]
  Bus 28/1 -> [v28]
  Bus 27/1 -> [v27]
  Bus 17/1 -> [v17]
  connections:
  Gen1/RConn3 -- Three-Phase Transformer (Two Windings)/LConn3
  Gen1/RConn2 -- Three-Phase Transformer (Two Windings)/LConn2
  Gen1/RConn1 -- Three-Phase Transformer (Two Windings)/LConn1
  Gen2/RConn1 -- Three-Phase Transformer (Two Windings)1/LConn1
  Gen2/RConn2 -- Three-Phase Transformer (Two Windings)1/LConn2
  Gen2/RConn3 -- Three-Phase Transformer (Two Windings)1/LConn3
  Gen3/RConn1 -- Three-Phase Transformer (Two Windings)2/LConn1
  Gen3/RConn2 -- Three-Phase Transformer (Two Windings)2/LConn2
  Gen3/RConn3 -- Three-Phase Transformer (Two Windings)2/LConn3
  Gen4/RConn1 -- Three-Phase Transformer (Two Windings)3/LConn1
  Gen4/RConn2 -- Three-Phase Transformer (Two Windings)3/LConn2
  Gen4/RConn3 -- Three-Phase Transformer (Two Windings)3/LConn3
  Gen5/RConn1 -- Three-Phase Transformer (Two Windings)4/LConn1
  Gen5/RConn2 -- Three-Phase Transformer (Two Windings)4/LConn2
  Gen5/RConn3 -- Three-Phase Transformer (Two Windings)4/LConn3
  Gen6/RConn1 -- Three-Phase Transformer (Two Windings)5/LConn1
  Gen6/RConn2 -- Three-Phase Transformer (Two Windings)5/LConn2
  Gen6/RConn3 -- Three-Phase Transformer (Two Windings)5/LConn3
  Three-Phase Series RLC Load1/LConn1 -- Bus 3/RConn1
  Three-Phase Series RLC Load1/LConn2 -- Bus 3/RConn2
  Three-Phase Series RLC Load1/LConn3 -- Bus 3/RConn3
  Three-Phase Series RLC Load2/LConn2 -- Bus 4/RConn2
  Three-Phase Series RLC Load2/LConn3 -- Bus 4/RConn3
  Three-Phase Series RLC Load2/LConn1 -- Bus 4/RConn1
  Three-Phase Series RLC Load5/LConn2 -- Bus 7/RConn2
  Three-Phase Series RLC Load5/LConn3 -- Bus 7/RConn3
  Three-Phase Series RLC Load5/LConn1 -- Bus 7/RConn1
  Three-Phase Series RLC Load7/LConn3 -- Bus 10/RConn3
  Three-Phase Series RLC Load7/LConn2 -- Bus 10/RConn2
  Three-Phase Series RLC Load7/LConn1 -- Bus 10/RConn1
  Three-Phase Series RLC Load9/LConn3 -- Bus 12/RConn3
  Three-Phase Series RLC Load9/LConn2 -- Bus 12/RConn2
  Three-Phase Series RLC Load9/LConn1 -- Bus 12/RConn1
  Three-Phase Series RLC Load10/LConn3 -- Bus 14/RConn3
  Three-Phase Series RLC Load10/LConn2 -- Bus 14/RConn2
  Three-Phase Series RLC Load10/LConn1 -- Bus 14/RConn1
  Three-Phase Series RLC Load11/LConn3 -- Bus 15/RConn3
  Three-Phase Series RLC Load11/LConn2 -- Bus 15/RConn2
  Three-Phase Series RLC Load11/LConn1 -- Bus 15/RConn1
  Three-Phase Transformer (Two Windings)/RConn1 -- Bus 1/RConn1
  Three-Phase Transformer (Two Windings)/RConn2 -- Bus 1/RConn2
  Three-Phase Transformer (Two Windings)/RConn3 -- Bus 1/RConn3
  Three-Phase Transformer (Two Windings)1/RConn1 -- Three-Phase Series RLC Load/LConn1 -- Three-Phase Fault/LConn1 -- Bus 2/RConn1
  Three-Phase Transformer (Two Windings)1/RConn2 -- Three-Phase Series RLC Load/LConn2 -- Three-Phase Fault/LConn2 -- Bus 2/RConn2
  Three-Phase Transformer (Two Windings)1/RConn3 -- Three-Phase Series RLC Load/LConn3 -- Three-Phase Fault/LConn3 -- Bus 2/RConn3
  Three-Phase Transformer (Two Windings)2/RConn1 -- Three-Phase Series RLC Load3/LConn1 -- Bus 5/RConn1
  Three-Phase Transformer (Two Windings)2/RConn2 -- Three-Phase Series RLC Load3/LConn2 -- Bus 5/RConn2
  Three-Phase Transformer (Two Windings)2/RConn3 -- Three-Phase Series RLC Load3/LConn3 -- Bus 5/RConn3
  Three-Phase Transformer (Two Windings)3/RConn1 -- Three-Phase Series RLC Load12/LConn1 -- Bus 8/RConn1
  Three-Phase Transformer (Two Windings)3/RConn2 -- Three-Phase Series RLC Load12/LConn2 -- Bus 8/RConn2
  Three-Phase Transformer (Two Windings)3/RConn3 -- Three-Phase Series RLC Load12/LConn3 -- Bus 8/RConn3
  Three-Phase Transformer (Two Windings)4/RConn1 -- Bus 11/RConn1
  Three-Phase Transformer (Two Windings)4/RConn2 -- Bus 11/RConn2
  Three-Phase Transformer (Two Windings)4/RConn3 -- Bus 11/RConn3
  Three-Phase Transformer (Two Windings)5/RConn1 -- Bus 13/RConn1
  Three-Phase Transformer (Two Windings)5/RConn2 -- Bus 13/RConn2
  Three-Phase Transformer (Two Windings)5/RConn3 -- Bus 13/RConn3
  Three-Phase Series RLC Branch/LConn1 -- Three-Phase Series RLC Branch1/LConn1 -- Bus 1/LConn1
  Three-Phase Series RLC Branch/LConn2 -- Three-Phase Series RLC Branch1/LConn2 -- Bus 1/LConn2
  Three-Phase Series RLC Branch/LConn3 -- Three-Phase Series RLC Branch1/LConn3 -- Bus 1/LConn3
  Three-Phase Series RLC Branch/RConn1 -- Three-Phase Series RLC Branch5/LConn1 -- Three-Phase Series RLC Branch4/LConn1 -- Three-Phase Series RLC Branch3/LConn1 -- Bus 2/LConn1
  Three-Phase Series RLC Branch/RConn2 -- Three-Phase Series RLC Branch5/LConn2 -- Three-Phase Series RLC Branch4/LConn2 -- Three-Phase Series RLC Branch3/LConn2 -- Bus 2/LConn2
  Three-Phase Series RLC Branch/RConn3 -- Three-Phase Series RLC Branch5/LConn3 -- Three-Phase Series RLC Branch4/LConn3 -- Three-Phase Series RLC Branch3/LConn3 -- Bus 2/LConn3
  Three-Phase Series RLC Branch1/RConn1 -- Three-Phase Series RLC Branch2/LConn1 -- Bus 3/LConn1
  Three-Phase Series RLC Branch1/RConn2 -- Three-Phase Series RLC Branch2/LConn2 -- Bus 3/LConn2
  Three-Phase Series RLC Branch1/RConn3 -- Three-Phase Series RLC Branch2/LConn3 -- Bus 3/LConn3
  Three-Phase Series RLC Branch2/RConn1 -- Three-Phase Series RLC Branch17/LConn1 -- Three-Phase Series RLC Branch3/RConn1 -- Three-Phase Series RLC Branch6/LConn1 -- Bus 4/LConn1
  Three-Phase Series RLC Branch2/RConn2 -- Three-Phase Series RLC Branch17/LConn2 -- Three-Phase Series RLC Branch3/RConn2 -- Three-Phase Series RLC Branch6/LConn2 -- Bus 4/LConn2
  Three-Phase Series RLC Branch2/RConn3 -- Three-Phase Series RLC Branch17/LConn3 -- Three-Phase Series RLC Branch3/RConn3 -- Three-Phase Series RLC Branch6/LConn3 -- Bus 4/LConn3
  Bus 5/LConn1 -- Three-Phase Series RLC Branch8/LConn1 -- Three-Phase Series RLC Branch4/RConn1
  Bus 5/LConn2 -- Three-Phase Series RLC Branch8/LConn2 -- Three-Phase Series RLC Branch4/RConn2
  Bus 5/LConn3 -- Three-Phase Series RLC Branch8/LConn3 -- Three-Phase Series RLC Branch4/RConn3
  Bus 6/LConn1 -- Three-Phase Series RLC Branch6/RConn1 -- Three-Phase Series RLC Branch9/LConn1 -- Three-Phase Series RLC Branch10/LConn1 -- Three-Phase Series RLC Branch5/RConn1 -- Three-Phase Series RLC Branch37/LConn1 -- Three-Phase Series RLC Branch12/LConn1
  Bus 6/LConn2 -- Three-Phase Series RLC Branch6/RConn2 -- Three-Phase Series RLC Branch9/LConn2 -- Three-Phase Series RLC Branch10/LConn2 -- Three-Phase Series RLC Branch12/LConn2 -- Three-Phase Series RLC Branch5/RConn2 -- Three-Phase Series RLC Branch37/LConn2
  Bus 6/LConn3 -- Three-Phase Series RLC Branch6/RConn3 -- Three-Phase Series RLC Branch9/LConn3 -- Three-Phase Series RLC Branch10/LConn3 -- Three-Phase Series RLC Branch12/LConn3 -- Three-Phase Series RLC Branch5/RConn3 -- Three-Phase Series RLC Branch37/LConn3
  Three-Phase Series RLC Branch7/RConn1 -- Bus 7/LConn1 -- Three-Phase Series RLC Branch8/RConn1
  Three-Phase Series RLC Branch7/RConn2 -- Three-Phase Series RLC Branch8/RConn2 -- Bus 7/LConn2
  Three-Phase Series RLC Branch7/RConn3 -- Three-Phase Series RLC Branch8/RConn3 -- Bus 7/LConn3
  Three-Phase Series RLC Branch9/RConn1 -- Three-Phase Series RLC Branch38/LConn1 -- Bus 8/LConn1
  Three-Phase Series RLC Branch9/RConn2 -- Bus 8/LConn2 -- Three-Phase Series RLC Branch38/LConn2
  Three-Phase Series RLC Branch9/RConn3 -- Three-Phase Series RLC Branch38/LConn3 -- Bus 8/LConn3
  Three-Phase Series RLC Branch10/RConn1 -- Three-Phase Series RLC Branch13/LConn1 -- Bus 9/LConn1
  Three-Phase Series RLC Branch10/RConn2 -- Three-Phase Series RLC Branch13/LConn2 -- Bus 9/LConn2
  Three-Phase Series RLC Branch10/RConn3 -- Three-Phase Series RLC Branch13/LConn3 -- Bus 9/LConn3
  Three-Phase Series RLC Branch11/LConn1 -- Bus 9/RConn1
  Three-Phase Series RLC Branch11/LConn2 -- Bus 9/RConn2
  Three-Phase Series RLC Branch11/LConn3 -- Bus 9/RConn3
  Three-Phase Series RLC Branch11/RConn1 -- Three-Phase Series RLC Branch12/RConn1 -- Three-Phase Series RLC Branch25/LConn1 -- Three-Phase Series RLC Branch27/RConn1 -- Three-Phase Series RLC Branch24/LConn1 -- Three-Phase Series RLC Branch20/LConn1 -- Bus 10/LConn1
  Three-Phase Series RLC Branch11/RConn2 -- Three-Phase Series RLC Branch12/RConn2 -- Three-Phase Series RLC Branch25/LConn2 -- Three-Phase Series RLC Branch27/RConn2 -- Three-Phase Series RLC Branch24/LConn2 -- Three-Phase Series RLC Branch20/LConn2 -- Bus 10/LConn2
  Three-Phase Series RLC Branch11/RConn3 -- Three-Phase Series RLC Branch12/RConn3 -- Three-Phase Series RLC Branch25/LConn3 -- Three-Phase Series RLC Branch27/RConn3 -- Three-Phase Series RLC Branch24/LConn3 -- Three-Phase Series RLC Branch20/LConn3 -- Bus 10/LConn3
  Three-Phase Series RLC Branch13/RConn1 -- Bus 11/LConn1
  Three-Phase Series RLC Branch13/RConn2 -- Bus 11/LConn2
  Three-Phase Series RLC Branch13/RConn3 -- Bus 11/LConn3
  Three-Phase Series RLC Branch14/LConn1 -- Three-Phase Series RLC Branch39/LConn1 -- Three-Phase Series RLC Branch18/LConn1 -- Three-Phase Series RLC Branch15/LConn1 -- Bus 12/LConn1
  Three-Phase Series RLC Branch14/LConn2 -- Three-Phase Series RLC Branch39/LConn2 -- Three-Phase Series RLC Branch18/LConn2 -- Three-Phase Series RLC Branch15/LConn2 -- Bus 12/LConn2
  Three-Phase Series RLC Branch14/LConn3 -- Three-Phase Series RLC Branch39/LConn3 -- Three-Phase Series RLC Branch18/LConn3 -- Three-Phase Series RLC Branch15/LConn3 -- Bus 12/LConn3
  Three-Phase Series RLC Branch14/RConn1 -- Bus 13/LConn1
  Three-Phase Series RLC Branch14/RConn2 -- Bus 13/LConn2
  Three-Phase Series RLC Branch14/RConn3 -- Bus 13/LConn3
  Three-Phase Series RLC Branch15/RConn1 -- Three-Phase Series RLC Branch16/LConn1 -- Bus 14/LConn1
  Three-Phase Series RLC Branch15/RConn2 -- Three-Phase Series RLC Branch16/LConn2 -- Bus 14/LConn2
  Three-Phase Series RLC Branch15/RConn3 -- Three-Phase Series RLC Branch16/LConn3 -- Bus 14/LConn3
  Three-Phase Series RLC Branch16/RConn1 -- Three-Phase Series RLC Branch39/RConn1 -- Three-Phase Series RLC Branch21/LConn1 -- Three-Phase Series RLC Branch28/LConn1 -- Three-Phase Series RLC Branch17/RConn1 -- Bus 15/LConn1
  Three-Phase Series RLC Branch16/RConn2 -- Three-Phase Series RLC Branch39/RConn2 -- Three-Phase Series RLC Branch21/LConn2 -- Three-Phase Series RLC Branch28/LConn2 -- Three-Phase Series RLC Branch17/RConn2 -- Bus 15/LConn2
  Three-Phase Series RLC Branch16/RConn3 -- Three-Phase Series RLC Branch39/RConn3 -- Three-Phase Series RLC Branch21/LConn3 -- Three-Phase Series RLC Branch28/LConn3 -- Three-Phase Series RLC Branch17/RConn3 -- Bus 15/LConn3
  Three-Phase Series RLC Load6/LConn1 -- Bus 16/LConn1
  Three-Phase Series RLC Load6/LConn2 -- Bus 16/LConn2
  Three-Phase Series RLC Load6/LConn3 -- Bus 16/LConn3
  Three-Phase Series RLC Load8/LConn1 -- Bus 17/LConn1
  Three-Phase Series RLC Load8/LConn2 -- Bus 17/LConn2
  Three-Phase Series RLC Load8/LConn3 -- Bus 17/LConn3
  Three-Phase Series RLC Load13/LConn1 -- Bus 18/LConn1
  Three-Phase Series RLC Load13/LConn2 -- Bus 18/LConn2
  Three-Phase Series RLC Load13/LConn3 -- Bus 18/LConn3
  Three-Phase Series RLC Load14/LConn1 -- Bus 19/LConn1
  Three-Phase Series RLC Load14/LConn2 -- Bus 19/LConn2
  Three-Phase Series RLC Load14/LConn3 -- Bus 19/LConn3
  Three-Phase Series RLC Load15/LConn1 -- Bus 20/LConn1
  Three-Phase Series RLC Load15/LConn2 -- Bus 20/LConn2
  Three-Phase Series RLC Load15/LConn3 -- Bus 20/LConn3
  Three-Phase Series RLC Load17/LConn1 -- Bus 23/LConn1
  Three-Phase Series RLC Load17/LConn2 -- Bus 23/LConn2
  Three-Phase Series RLC Load17/LConn3 -- Bus 23/LConn3
  Three-Phase Series RLC Load18/LConn1 -- Bus 24/LConn1
  Three-Phase Series RLC Load18/LConn2 -- Bus 24/LConn2
  Three-Phase Series RLC Load18/LConn3 -- Bus 24/LConn3
  Three-Phase Series RLC Load19/LConn1 -- Bus 26/LConn1
  Three-Phase Series RLC Load19/LConn2 -- Bus 26/LConn2
  Three-Phase Series RLC Load19/LConn3 -- Bus 26/LConn3
  Three-Phase Series RLC Load21/LConn1 -- Bus 29/LConn1
  Three-Phase Series RLC Load21/LConn2 -- Bus 29/LConn2
  Three-Phase Series RLC Load21/LConn3 -- Bus 29/LConn3
  Three-Phase Series RLC Load22/LConn1 -- Bus 30/LConn1
  Three-Phase Series RLC Load22/LConn2 -- Bus 30/LConn2
  Three-Phase Series RLC Load22/LConn3 -- Bus 30/LConn3
  Three-Phase Series RLC Branch18/RConn1 -- Three-Phase Series RLC Branch19/LConn1 -- Three-Phase Series RLC Branch19/LConn2 -- Three-Phase Series RLC Branch19/LConn3 -- Bus 16/RConn1
  Three-Phase Series RLC Branch18/RConn2 -- Bus 16/RConn2
  Three-Phase Series RLC Branch18/RConn3 -- Bus 16/RConn3
  Three-Phase Series RLC Branch19/RConn1 -- Three-Phase Series RLC Branch20/RConn1 -- Bus 17/RConn1
  Three-Phase Series RLC Branch19/RConn2 -- Three-Phase Series RLC Branch20/RConn2 -- Bus 17/RConn2
  Three-Phase Series RLC Branch19/RConn3 -- Three-Phase Series RLC Branch20/RConn3 -- Bus 17/RConn3
  Three-Phase Series RLC Branch21/RConn1 -- Bus 18/RConn1 -- Three-Phase Series RLC Branch22/LConn1
  Three-Phase Series RLC Branch21/RConn2 -- Bus 18/RConn2 -- Three-Phase Series RLC Branch22/LConn2
  Three-Phase Series RLC Branch21/RConn3 -- Bus 18/RConn3 -- Three-Phase Series RLC Branch22/LConn3
  Three-Phase Series RLC Branch22/RConn1 -- Bus 19/RConn1 -- Three-Phase Series RLC Branch23/LConn1
  Three-Phase Series RLC Branch22/RConn2 -- Bus 19/RConn2 -- Three-Phase Series RLC Branch23/LConn2
  Three-Phase Series RLC Branch22/RConn3 -- Bus 19/RConn3 -- Three-Phase Series RLC Branch23/LConn3
  Three-Phase Series RLC Branch23/RConn1 -- Bus 20/RConn1 -- Three-Phase Series RLC Branch24/RConn1
  Three-Phase Series RLC Branch23/RConn2 -- Bus 20/RConn2 -- Three-Phase Series RLC Branch24/RConn2
  Three-Phase Series RLC Branch23/RConn3 -- Bus 20/RConn3 -- Three-Phase Series RLC Branch24/RConn3
  Three-Phase Series RLC Load16/LConn3 -- Bus 21/LConn3
  Three-Phase Series RLC Load16/LConn2 -- Bus 21/LConn2
  Three-Phase Series RLC Load16/LConn1 -- Bus 21/LConn1
  Three-Phase Series RLC Branch25/RConn1 -- Bus 21/RConn1 -- Three-Phase Series RLC Branch26/LConn1
  Three-Phase Series RLC Branch25/RConn2 -- Bus 21/RConn2 -- Three-Phase Series RLC Branch26/LConn2
  Three-Phase Series RLC Branch25/RConn3 -- Bus 21/RConn3 -- Three-Phase Series RLC Branch26/LConn3
  Three-Phase Series RLC Branch26/RConn1 -- Bus 22/RConn1 -- Three-Phase Series RLC Branch29/LConn1
  Three-Phase Series RLC Branch26/RConn2 -- Bus 22/RConn2 -- Three-Phase Series RLC Branch29/LConn2
  Three-Phase Series RLC Branch26/RConn3 -- Bus 22/RConn3 -- Three-Phase Series RLC Branch29/LConn3
  Three-Phase Series RLC Branch28/RConn1 -- Three-Phase Series RLC Branch30/LConn1 -- Bus 23/RConn1
  Three-Phase Series RLC Branch28/RConn2 -- Three-Phase Series RLC Branch30/LConn2 -- Bus 23/RConn2
  Three-Phase Series RLC Branch28/RConn3 -- Three-Phase Series RLC Branch30/LConn3 -- Bus 23/RConn3
  Three-Phase Series RLC Branch29/RConn1 -- Three-Phase Series RLC Branch31/LConn1 -- Three-Phase Series RLC Branch30/RConn1 -- Bus 24/RConn1
  Three-Phase Series RLC Branch29/RConn2 -- Three-Phase Series RLC Branch31/LConn2 -- Three-Phase Series RLC Branch30/RConn2 -- Bus 24/RConn2
  Three-Phase Series RLC Branch29/RConn3 -- Three-Phase Series RLC Branch31/LConn3 -- Three-Phase Series RLC Branch30/RConn3 -- Bus 24/RConn3
  Three-Phase Series RLC Branch31/RConn1 -- Bus 25/RConn1
  Three-Phase Series RLC Branch31/RConn2 -- Bus 25/RConn2
  Three-Phase Series RLC Branch31/RConn3 -- Bus 25/RConn3
  Three-Phase Series RLC Branch32/LConn1 -- Three-Phase Series RLC Branch33/LConn1 -- Bus 25/LConn1
  Bus 25/LConn2 -- Three-Phase Series RLC Branch32/LConn2 -- Three-Phase Series RLC Branch33/LConn2
  Three-Phase Series RLC Branch32/LConn3 -- Three-Phase Series RLC Branch33/LConn3 -- Bus 25/LConn3
  Three-Phase Series RLC Branch32/RConn1 -- Bus 26/RConn1
  Three-Phase Series RLC Branch32/RConn2 -- Bus 26/RConn2
  Three-Phase Series RLC Branch32/RConn3 -- Bus 26/RConn3
  Three-Phase Series RLC Branch35/LConn1 -- Three-Phase Series RLC Branch34/LConn1 -- Three-Phase Series RLC Branch36/RConn1 -- Bus 27/RConn1
  Three-Phase Series RLC Branch35/LConn2 -- Three-Phase Series RLC Branch34/LConn2 -- Three-Phase Series RLC Branch36/RConn2 -- Bus 27/RConn2
  Three-Phase Series RLC Branch35/LConn3 -- Three-Phase Series RLC Branch34/LConn3 -- Three-Phase Series RLC Branch36/RConn3 -- Bus 27/RConn3
  Three-Phase Series RLC Branch34/RConn1 -- Three-Phase Series RLC Branch40/LConn1 -- Bus 29/RConn1
  Three-Phase Series RLC Branch34/RConn2 -- Three-Phase Series RLC Branch40/LConn2 -- Bus 29/RConn2
  Three-Phase Series RLC Branch34/RConn3 -- Three-Phase Series RLC Branch40/LConn3 -- Bus 29/RConn3
  Three-Phase Series RLC Branch35/RConn1 -- Three-Phase Series RLC Branch40/RConn1 -- Bus 30/RConn1
  Three-Phase Series RLC Branch35/RConn2 -- Three-Phase Series RLC Branch40/RConn2 -- Bus 30/RConn2
  Three-Phase Series RLC Branch35/RConn3 -- Three-Phase Series RLC Branch40/RConn3 -- Bus 30/RConn3
  Bus 28/LConn1 -- Three-Phase Series RLC Branch36/LConn1
  Bus 28/LConn2 -- Three-Phase Series RLC Branch36/LConn2
  Bus 28/LConn3 -- Three-Phase Series RLC Branch36/LConn3
  Bus 28/RConn1 -- Three-Phase Series RLC Branch38/RConn1 -- Three-Phase Series RLC Branch37/RConn1
  Bus 28/RConn2 -- Three-Phase Series RLC Branch38/RConn2 -- Three-Phase Series RLC Branch37/RConn2
  Bus 28/RConn3 -- Three-Phase Series RLC Branch38/RConn3 -- Three-Phase Series RLC Branch37/RConn3
  Three-Phase Series RLC Branch27/LConn2 -- Bus 22/LConn2
  Bus 22/LConn3 -- Three-Phase Series RLC Branch27/LConn3
  Bus 22/LConn1 -- Three-Phase Series RLC Branch27/LConn1
  Three-Phase Series RLC Branch7/LConn1 -- Bus 6/RConn1
  Three-Phase Series RLC Branch7/LConn2 -- Bus 6/RConn2
  Three-Phase Series RLC Branch7/LConn3 -- Bus 6/RConn3
  Three-Phase Series RLC Branch33/RConn1 -- Bus 27/LConn1
  Three-Phase Series RLC Branch33/RConn2 -- Bus 27/LConn2
  Three-Phase Series RLC Branch33/RConn3 -- Bus 27/LConn3
